simulink model "path_estimation_test"  (R2023b)
settings: Solver=ode3  StartTime=0.0  StopTime=5  RelTol=1e-3  EnableMultiTasking=on
libraries: audiosources x2, dspadpt3 x1
settings Model: FPTRunName=Active  ExtModeTrigDuration=2  Creator=aaron  LastModifiedBy=aaron
settings SolverCC: AlgebraicLoopSolver=TrustRegion  PositivePriorityOrder=on
settings DataIOCC: LimitDataPoints=on  SaveFormat=Array
settings OptimizationCC: ExpressionDepthLimit=2147483647  LifeSpan=Inf  MaxStackSize=64
settings DebuggingCC: ReadBeforeWriteMsg=DisableAll  WriteAfterWriteMsg=DisableAll  WriteAfterReadMsg=DisableAll  UnderspecifiedInitializationDetection=Classic  MergeDetectMultiDrivingBlocksExec=none  MultiTaskDSMMsg=none  FcnCallInpInsideContextMsg=warning  UnconnectedInputMsg=warning  UnconnectedOutputMsg=warning  UnconnectedLineMsg=warning  AllowSymbolicDim=off  StateNameClashWarn=warning  SubsystemReferenceDiagnosticForUnitTest=warning  SFUnexpectedBacktrackingDiag=warning  SFNoUnconditionalDefaultTransitionDiag=warning  SFExecutionAtInitializationDiag=none  ArithmeticOperatorsInVariantConditions=warning
settings HardwareCC: ProdBitPerPointer=32  ProdBitPerSizeT=32  ProdBitPerPtrDiffT=32  ProdLargestAtomicInteger=Long  ProdLargestAtomicFloat=Double  ProdWordSize=32  ProdHWDeviceType=ARM Compatible->ARM Cortex  UseEmbeddedCoderFeatures=off  UseSimulinkCoderFeatures=off
settings ModelReferenceCC: UpdateModelReferenceTargets=IfOutOfDate  EnableRefExpFcnMdlSchedulingChecks=on  PropagateSignalLabelsOutOfModel=off
settings SFSimCC: SFSimEcho=off  SimUseLocalCustomCode=off  CustomCodeUndefinedFunction=UseInterfaceOnly
settings RTWCC: Description=Embedded Coder  SystemTargetFile=ert.tlc  HardwareBoard=Raspberry Pi  TemplateMakefile=ert_default_tmf  GenerateReport=on  RTWVerbose=off  RTWUseLocalCustomCode=off  Toolchain=GNU GCC Embedded Linux  BuildConfiguration=Faster Runs  LaunchReport=on
settings CodeAppCC: ForceParamTrailComments=on  OperatorAnnotations=on  StateflowObjectComments=on  MATLABSourceComments=on
settings ERTTargetCC: MultiwordLength=2048  ERTCustomFileBanners=off  SupportContinuousTime=on  SupportNonInlinedSFcns=on  RemoveResetFunc=off  SupportVariableSizeSignals=on  ModelStepFunctionPrototypeControlCompliant=off
settings ConfigComp: CovMetricSettings=dw  CovSaveCumulativeToWorkspaceVar=on  CovSaveSingleToWorkspaceVar=on  CovExternalEMLEnable=off  CovSFcnEnable=off

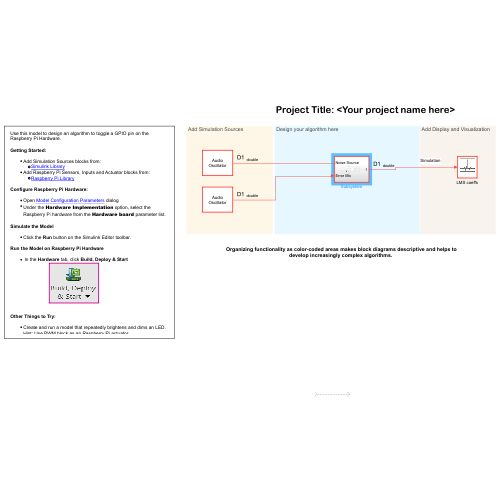
[thumbnail: Simulink's stored preview of the top-level diagram]
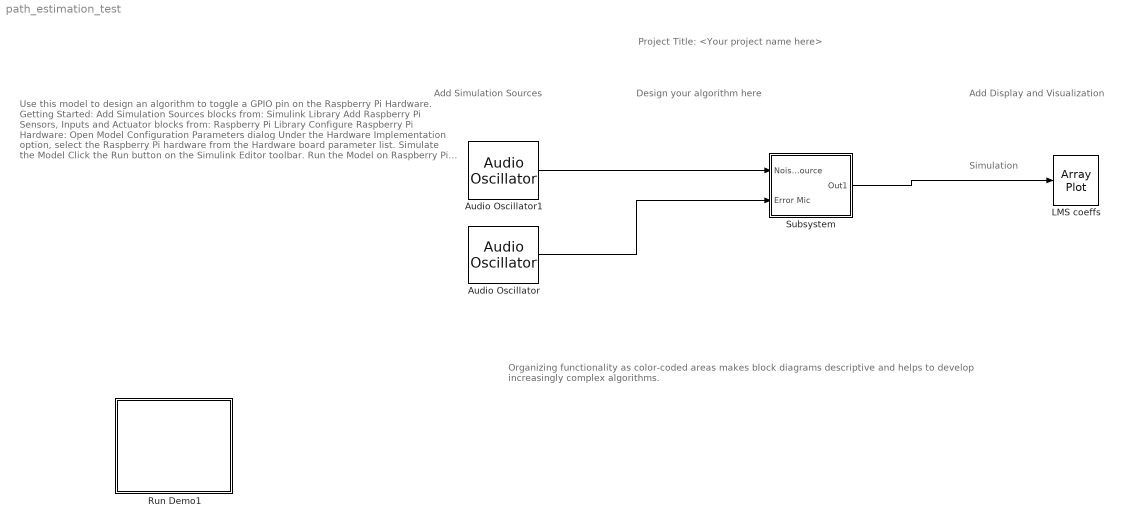
== system path_estimation_test ==
  note: Simulation
  note: Add Simulation Sources
  note: Project Title: <Your project name here>
  note: Organizing functionality as color-coded areas makes block diagrams descriptive and helps to develop increasingly complex algorithms.
  note: Design your algorithm here
  note: Add Display and Visualization
  note: Use this model to design an algorithm to toggle a GPIO pin on the Raspberry Pi Hardware.
      |
      | Getting Started:
      |
      | Add Simulation Sources blocks from:
      | Simulink Library
      | Add Raspberry Pi Sensors, Inputs and Actuator blocks from:
      | Raspberry Pi Library
      |
      | Configure Raspberry Pi Hardware:
      |
      | Open Model Configuration Parameters dialog
      | Under the Hardware Implementation option, select the Raspberry Pi hardware from the Hardware board parameter list.
      |
      | Simulate the Model
      |
      | Click the Run button on the Simulink Editor toolbar.
      |
      | Run the Model on Raspberry Pi Hardware
      |
      | In the Hardware tab, click Build, Deploy & Start
      |
      | Other Things to Try:
      |
      | Create and run a model that repeatedly brightens and dims an LED. Hint: Use PWM block as an Raspberry Pi actuator.
  Audio Oscillator : audiosources/Audio Oscillator  FrequencyPort=off  Frequency=300  AmplitudePort=off  Amplitude=30000  DCOffsetPort=off  PhaseOffset=0.9  DCOffset=0  WidthPort=off  Width=1  DutyCyclePort=off  DutyCycle=0.5  SampsPerFrame=1  Fs=44100  OutputDataType=double  SimulateUsing=Interpreted execution
      settings: SignalType=sine
  Audio Oscillator1 : audiosources/Audio Oscillator  FrequencyPort=off  Frequency=300  AmplitudePort=off  Amplitude=30000  DCOffsetPort=off  PhaseOffset=0  DCOffset=0  WidthPort=off  Width=1  DutyCyclePort=off  DutyCycle=0.5  SampsPerFrame=1  Fs=44100  OutputDataType=double  SimulateUsing=Interpreted execution
      settings: SignalType=sine
  LMS coeffs : ArrayPlot  WindowPosition=[27.000000,288.000000,800.000000,500.000000,]  ScopeFrameLocation=window  AxesScaling=Manual  YLimits=[0 10]  DefaultConfigurationName=dsp.scopes.ArrayPlotBlockSpecification
  Run Demo1 : Subsystem  Description=Controls host-side RTDX processing.
      mask Display: pic=imread('raspberrypiBuildDeployAndStart.png');image(pic);
  Subsystem : Subsystem
  wires:
  ? -> ?
  Audio Oscillator1/1 -> Subsystem/1(Noise Source)
  Subsystem/1(Out1) -> LMS coeffs/1
  Audio Oscillator/1 -> Subsystem/2(Error Mic)

== system path_estimation_test/Run Demo1 ==

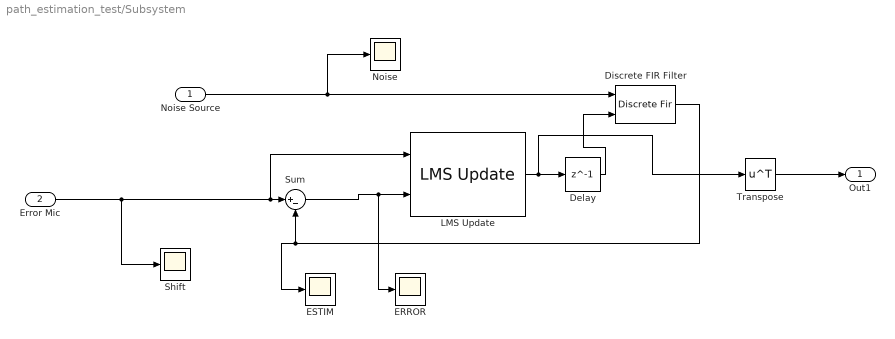
== system path_estimation_test/Subsystem ==
  Noise Source : Inport
  Error Mic : Inport  Port=2
  Delay : Delay  DelayLength=1  InitialCondition=0
  Discrete FIR Filter : DiscreteFir  CoefSource=Input port
      settings: InputPortMap=u0,u1
  ERROR : Scope
  ESTIM : Scope
  LMS Update : dspadpt3/LMS Update  Method=Normalized LMS  Length=32  NumFilters=1  StepSizeSource=Property  StepSize=0.1  LeakageFactor=1  InitialConditions=0  AdaptiveFilterMode=Tapped delay-line FIR filter  EnableAdaptInput=off  EnableResetInput=off  SimulateUsing=Interpreted execution
  Noise : Scope
  Shift : Scope
  Sum : Sum  Inputs=|+-
  Transpose : Math  Operator=transpose
  Out1 : Outport
  wires:
  LMS Update/1 -> Transpose/1, Delay/1
  Sum/1 -> ERROR/1, LMS Update/2
  Noise Source/1 -> Noise/1, Discrete FIR Filter/1
  Delay/1 -> Discrete FIR Filter/2
  Discrete FIR Filter/1 -> ESTIM/1, Sum/2
  Transpose/1 -> Out1/1
  Error Mic/1 -> Shift/1, LMS Update/1, Sum/1
